simulink model "simulinkPartB"  (R2017b)
settings: Solver=VariableStepAuto  StartTime=0.0  StopTime=10.0  RelTol=1e-3
settings Model: Creator=Vian  LastModifiedBy=Vian

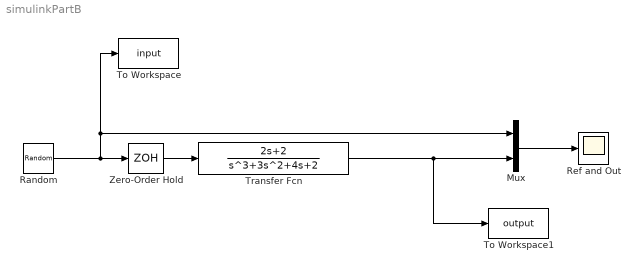
== system simulinkPartB ==
  Mux : Mux  Inputs=2
  Random : RandomNumber  SampleTime=0.1
  "Ref and Out " : Scope
  To Workspace : ToWorkspace  VariableName=input  SaveFormat=Timeseries  SampleTime=-1
  To Workspace1 : ToWorkspace  VariableName=output  SaveFormat=Timeseries  SampleTime=-1
  Transfer Fcn : TransferFcn  Numerator=[2 2]  Denominator=[1 3 4 2]
  Zero-Order Hold : ZeroOrderHold  SampleTime=0.1
  wires:
  Random/1 -> To Workspace/1, Mux/1, Zero-Order Hold/1
  Zero-Order Hold/1 -> Transfer Fcn/1
  Mux/1 -> "Ref and Out "/1
  Transfer Fcn/1 -> To Workspace1/1, Mux/2
